simulink subsystem "MotorsDCFaulhaber"  (R2023b)
settings: Solver=VariableStepAuto  StartTime=0.0  StopTime=10.0  RelTol=1e-3
undefined symbols (not defined in the file): Motor1_C, Motor1_Neg, Motor1_Pos, Motor1_R, Motor2_C, Motor2_Neg, Motor2_Pos, Motor2_R, Motor3_C, Motor3_Neg, Motor3_Pos, Motor3_R
settings Model: DataDictionary=neck_mk3.sldd  EnableAccessToBaseWorkspace=off  Creator=upattacini  LastModifiedBy=upattacini

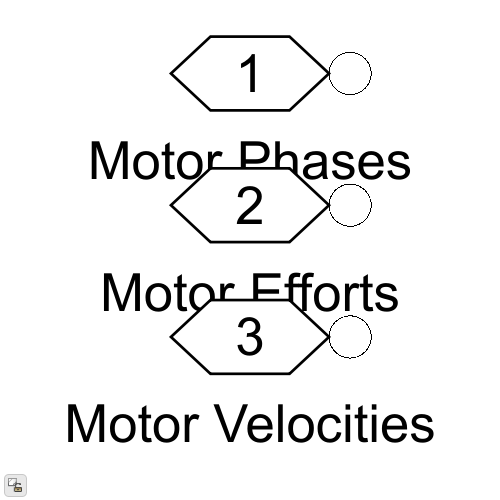
[thumbnail: Simulink's stored preview of the top-level diagram]
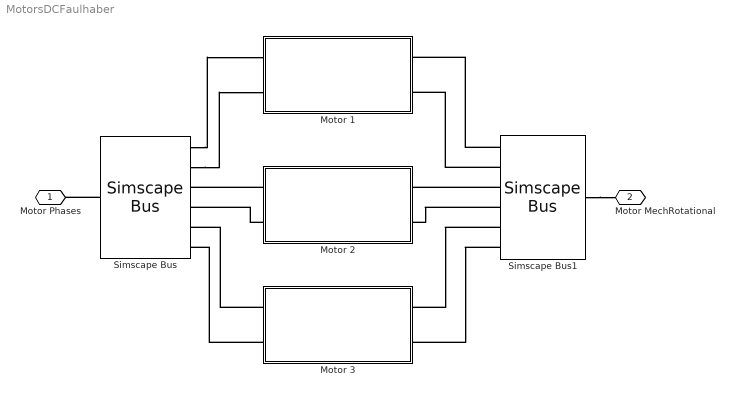
== system MotorsDCFaulhaber ==
  Motor 1 : Subsystem  ReferencedSubsystem=DCFaulhaber
      settings: PermitHierarchicalResolution=None
  Motor 2 : Subsystem  ReferencedSubsystem=DCFaulhaber
      settings: PermitHierarchicalResolution=None
  Motor 3 : Subsystem  ReferencedSubsystem=DCFaulhaber
      settings: PermitHierarchicalResolution=None
  Simscape Bus : SimscapeBus  HierarchyStrings=Motor1_Pos;Motor1_Neg;Motor2_Pos;Motor2_Neg;Motor3_Pos;Motor3_Neg  ConnectionType=Bus: Physical_Phases
  Simscape Bus1 : SimscapeBus  HierarchyStrings=Motor1_R;Motor1_C;Motor2_R;Motor2_C;Motor3_R;Motor3_C  ConnectionType=Bus: Physical_MechRotationals
  Motor Phases : PMIOPort  Side=Left
  Motor MechRotational : PMIOPort  Port=2  Side=Right
  connections:
  Simscape Bus/RConn1 -- Motor Phases/RConn1
  Simscape Bus/LConn1 -- Motor 1/LConn1
  Simscape Bus/LConn2 -- Motor 1/LConn2
  Motor 2/LConn1 -- Simscape Bus/LConn3
  Motor 2/LConn2 -- Simscape Bus/LConn4
  Motor 3/LConn1 -- Simscape Bus/LConn5
  Motor 3/LConn2 -- Simscape Bus/LConn6
  Simscape Bus1/LConn1 -- Motor 1/RConn1
  Simscape Bus1/LConn2 -- Motor 1/RConn2
  Simscape Bus1/LConn3 -- Motor 2/RConn1
  Simscape Bus1/LConn4 -- Motor 2/RConn2
  Simscape Bus1/LConn5 -- Motor 3/RConn1
  Simscape Bus1/LConn6 -- Motor 3/RConn2
  Simscape Bus1/RConn1 -- Motor MechRotational/RConn1
